simulink model "mux"  (R2020a)
settings: Solver=VariableStepAuto  StartTime=0.0  StopTime=10.0  RelTol=1e-3
settings Model: Creator=Administrator  LastModifiedBy=Administrator

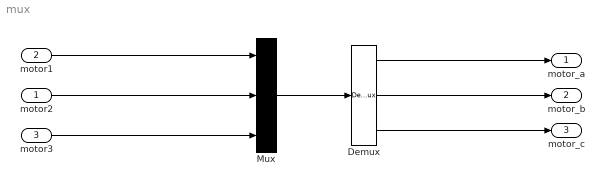
== system mux ==
  motor2 : Inport
  motor1 : Inport  Port=2
  motor3 : Inport  Port=3
  Demux : Demux  Outputs=3
  Mux : Mux  Inputs=3
  motor_a : Outport
  motor_b : Outport  Port=2
  motor_c : Outport  Port=3
  wires:
  motor1/1 -> Mux/1
  motor2/1 -> Mux/2
  motor3/1 -> Mux/3
  Demux/1 -> motor_a/1
  Demux/2 -> motor_b/1
  Demux/3 -> motor_c/1
  Mux/1 -> Demux/1
